simulink model "UAV"  (R2021b)
settings: Solver=ode45  StartTime=0.0  StopTime=10000  RelTol=1e-3
InitFcn:
  | param
values from neighbouring files (symbols this model uses):
  P = [-0.6408, 0.37, 0.6408, -0.37; -0.37, -0.6408, 0.37, 0.6408; 0.002*((s+0.1)^2), 0.002*((s+0.1)^2), 0.002*((s+0.1)^2), 0.002*((s+0.1)^2); -0.25*((s+0.1)^2), 0.25*((s+0.1)^2), -0.25*((s+0.1)^2), 0.25*((s+0.1)^2)]    [quadrotor_plant.m]    (also in youla_controller.m; youlascripts.m = [-0.6408, 0.37, 0.6408, -0.37; -0.37, -0.6408, 0.37, 0.6408;)
undefined symbols (not defined in the file or in its folder): forces_moments
settings Model: Creator=beard  LastModifiedBy=yuankaizhu
settings SolverCC: AlgebraicLoopSolver=TrustRegion
settings DataIOCC: LimitDataPoints=on  SaveFormat=Array  ReturnWorkspaceOutputs=off
settings OptimizationCC: BlockReduction=off  BooleanDataType=off  LifeSpan=inf
settings DebuggingCC: SaveWithParameterizedLinksMsg=none  UnderspecifiedInitializationDetection=Classic  MergeDetectMultiDrivingBlocksExec=none  SignalResolutionControl=TryResolveAllWithWarning  SFUnexpectedBacktrackingDiag=warning  SFNoUnconditionalDefaultTransitionDiag=warning  SFExecutionAtInitializationDiag=none  SFMachineParentedDataDiag=warning  ArithmeticOperatorsInVariantConditions=warning
settings HardwareCC: ProdBitPerPointer=32  ProdBitPerSizeT=32  ProdBitPerPtrDiffT=32  ProdLargestAtomicFloat=None  ProdIntDivRoundTo=Undefined  ProdEndianess=Unspecified  ProdWordSize=32  ProdHWDeviceType=32-bit Generic  TargetUnknown=on
settings ModelReferenceCC: PropagateSignalLabelsOutOfModel=off
settings SFSimCC: SimUseLocalCustomCode=off  CustomCodeUndefinedFunction=UseInterfaceOnly
settings RTWCC: RTWUseLocalCustomCode=off
settings CodeAppCC: StateflowObjectComments=on
settings GRTTargetCC: TargetLangStandard=C89/C90 (ANSI)
settings ConfigComp: CovMetricSettings=dw  CovSaveCumulativeToWorkspaceVar=on  CovSaveSingleToWorkspaceVar=on  CovExternalEMLEnable=off  CovSFcnEnable=off

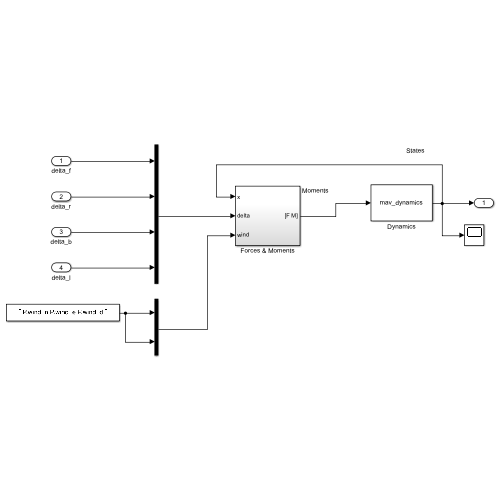
[thumbnail: Simulink's stored preview of the top-level diagram]
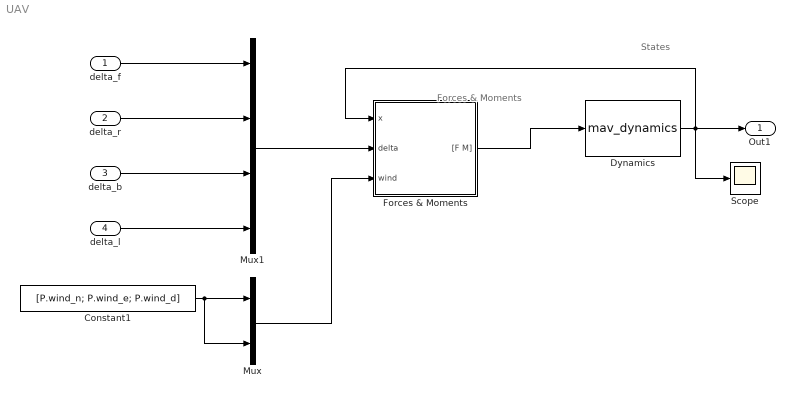
== system UAV ==
  note: Forces & Moments
  note: States
  delta_f : Inport
  delta_r : Inport  Port=2
  delta_b : Inport  Port=3
  delta_l : Inport  Port=4
  Constant1 : Constant  Value=[P.wind_n; P.wind_e; P.wind_d]
  Dynamics : S-Function  FunctionName=mav_dynamics  Parameters=P,0  SFunctionDeploymentMode=off  EnableBusSupport=off
  Forces & Moments : Subsystem
  Mux : Mux  Inputs=2
  Mux1 : Mux
  Scope : Scope
  Out1 : Outport
  wires:
  Dynamics/1 -> Scope/1, Out1/1, Forces & Moments/1(x)
  delta_l/1 -> Mux1/4
  Mux1/1 -> Forces & Moments/2(delta)
  Forces & Moments/1("[F M]") -> Dynamics/1
  Mux/1 -> Forces & Moments/3(wind)
  Constant1/1 -> Mux/2, Mux/1
  delta_f/1 -> Mux1/1
  delta_r/1 -> Mux1/2
  delta_b/1 -> Mux1/3

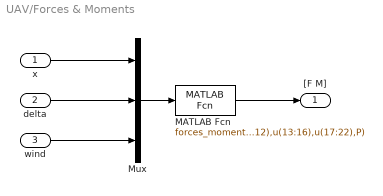
== system UAV/Forces & Moments ==
  x : Inport
  delta : Inport  Port=2
  wind : Inport  Port=3
  MATLAB Fcn : MATLABFcn  MATLABFcn=forces_moments(u(1:12),u(13:16),u(17:22),P)  OutputDimensions=6
  Mux : Mux  Inputs=3
  "[F M]" : Outport
  wires:
  x/1 -> Mux/1
  delta/1 -> Mux/2
  wind/1 -> Mux/3
  MATLAB Fcn/1 -> "[F M]"/1
  Mux/1 -> MATLAB Fcn/1
